simulink model "Totem_PSFB_Charger"  (R2022a)
settings: Solver=ode4  StartTime=0.0  StopTime=1  FixedStep=1e-7  RelTol=1e-3
undefined symbols (not defined in the file): C_PSFB, C_totem, fs_PFC, Gci_inf, Gcinf, Gcv_inf, Gcvinf, H, H_PSFB, kx, L_PSFB, L_totem, Rsense, Rsense_PSFB, Vm, wL, wLi_PSFB, wLv_PSFB, wLvv
libraries: spsMosfetLib x9, spsDiodeLib x8, spsSeriesRLCBranchLib x8, spsVoltageMeasurementLib x4, spsCurrentMeasurementLib x2, spsACVoltageSourceLib x1, hdlsllib x1, spsLinearTransformerLib x1, spsDCVoltageSourceLib x1, spsRMSLib x1, simulink x1, spspowerguiLib x1
settings Model: Creator=Aditya Bhalotia  LastModifiedBy=Aditya Bhalotia
settings DataIOCC: ReturnWorkspaceOutputs=off

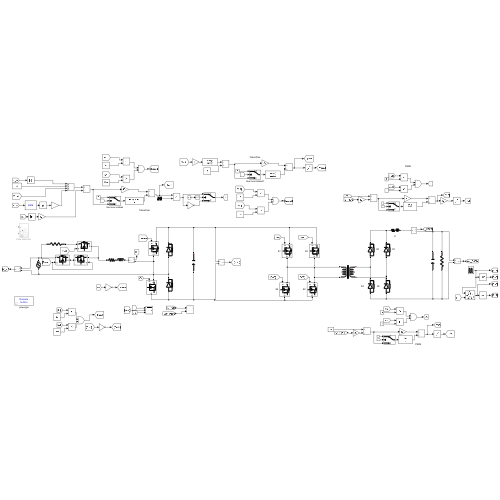
[thumbnail: Simulink's stored preview of the top-level diagram]
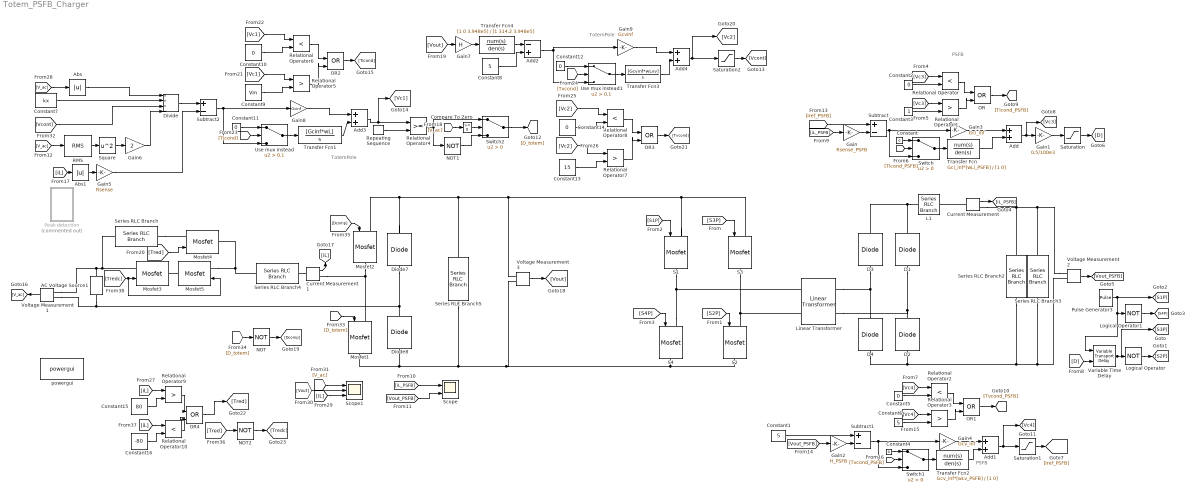
== system Totem_PSFB_Charger ==
  note: TotemPole
  note: PSFB
  note: PSFB
  note: TotemPole
  AC Voltage Source1 : spsACVoltageSourceLib/AC Voltage Source  Amplitude=265*sqrt(2)  Phase=0  Frequency=65  SampleTime=0  Measurements=None  BusType=swing  Pref=10e3  Qref=0  Qmin=-inf  Qmax=+inf
  Abs : Abs  SaturateOnIntegerOverflow=off
  Abs1 : Abs  SaturateOnIntegerOverflow=off
  Add{,1,3..4} (4 alike) : Sum
  Add2 : Sum  Inputs=-+
  Compare To Zero : hdlsllib/Logic and Bit Operations/Compare To Zero  relop=>=  OutDataTypeStr=boolean
      settings: SourceProductBaseCode=SL
  Constant{,2,4..5,10..12,14} (8 alike) : Constant  Value=0
  Constant1 : Constant  Value=5
  Constant13 : Constant  Value=15
  Constant15 : Constant  Value=80
  Constant16 : Constant  Value=-80
  Constant3 : Constant
  Constant6 : Constant  Value=5
  Constant7 : Constant  Value=kx
  Constant8 : Constant  Value=5
  Constant9 : Constant  Value=Vm
  Current Measurement : spsCurrentMeasurementLib/Current Measurement  PhasorSimulation=off  OutputType=Complex  PSBequivalent=0
  Current Measurement1 : spsCurrentMeasurementLib/Current Measurement  PhasorSimulation=off  OutputType=Complex  PSBequivalent=0
  D{1..4} (4 alike) : spsDiodeLib/Diode  Ron=0.001  Lon=0  Vf=1  IC=0  UseSnubber=0  Rs=500e6  Cs=1e-15  Measurements=off
  Diode7 : spsDiodeLib/Diode  Ron=0.001  Lon=0  Vf=0  IC=0  UseSnubber=0  Rs=50e3  Cs=inf  Measurements=off
  Diode8 : spsDiodeLib/Diode  Ron=0.001  Lon=0  Vf=0  IC=0  UseSnubber=0  Rs=50e3  Cs=inf  Measurements=off
  Divide : Product  Inputs=***/
  Gain : Gain  Gain=Rsense_PSFB
  Gain1 : Gain  Gain=0.5/100e3
  Gain2 : Gain  Gain=H_PSFB
  Gain3 : Gain  Gain=Gci_inf
  Gain4 : Gain  Gain=Gcv_inf
  Gain5 : Gain  Gain=Rsense
  Gain6 : Gain  Gain=2
  Gain7 : Gain  Gain=H
  Gain8 : Gain  Gain=Gcinf
  Gain9 : Gain  Gain=Gcvinf
  L1 : spsSeriesRLCBranchLib/Series RLC Branch  LConnTagsString=__new0  RConnTagsString=__new0  BranchType=RL  Resistance=0.1  Inductance=L_PSFB  SetiL0=off  InitialCurrent=0  Capacitance=1e-6  Setx0=off  InitialVoltage=0  Measurements=Branch current
  Linear Transformer : spsLinearTransformerLib/Linear Transformer  UNITS=SI  NominalPower=[50e2 100e3]  winding1=[400 0.01 0]  winding2=[400 0.01 0]  ThreeWindings=off  winding3=[3.15e+05 0.7938 0.084225]  RmLm=[1.0804e5 28e-3]  Measurements=None  DataType=on
  Logical Operator : Logic  Operator=NOT  AllPortsSameDT=off  OutDataTypeStr=boolean
  Logical Operator1 : Logic  Operator=NOT  AllPortsSameDT=off  OutDataTypeStr=boolean
  Mosfet{1..5} (5 alike) : spsMosfetLib/Mosfet  Ron=0.0001  Lon=0  Rd=0.0001  Vfd=0  IC=0  Rs=50e4  Cs=inf  Measurements=off
  NOT : Logic  Operator=NOT  IconShape=distinctive  AllPortsSameDT=off  OutDataTypeStr=boolean
  NOT1 : Logic  Operator=NOT  IconShape=distinctive  AllPortsSameDT=off  OutDataTypeStr=boolean
  NOT2 : Logic  Operator=NOT  IconShape=distinctive  AllPortsSameDT=off  OutDataTypeStr=boolean
  OR{,1..4} (5 alike) : Logic  Operator=OR  IconShape=distinctive  AllPortsSameDT=off  OutDataTypeStr=boolean
  Peak detection : Subsystem  Commented=on
  Pulse Generator3 : DiscretePulseGenerator  PulseType=Time based  Period=10e-6  PulseWidth=50
  RMS : spsRMSLib/RMS  TrueRMS=off  Freq=65  RMSInit=220  Ts=0
  Relational Operator{,2,6,8,10} (5 alike) : RelationalOperator  Operator=<  OutDataTypeStr=boolean  RndMeth=Simplest  InputSameDT=off
  Relational Operator{1,3,5,7,9} (5 alike) : RelationalOperator  Operator=>  OutDataTypeStr=boolean  RndMeth=Simplest  InputSameDT=off
  Relational Operator4 : RelationalOperator  OutDataTypeStr=boolean  RndMeth=Simplest  InputSameDT=off
  Repeating Sequence : simulink/Sources/Repeating Sequence  rep_seq_t=[0 1/fs_PFC]  rep_seq_y=[0 Vm]
  S{1..4} (4 alike) : spsMosfetLib/Mosfet  Ron=0.001  Lon=0  Rd=0.01  Vfd=0  IC=0  Rs=1e5  Cs=inf  Measurements=off
  Saturation : Saturate  UpperLimit=5e-6  LowerLimit=0
  Saturation1 : Saturate  UpperLimit=5  LowerLimit=0
  Saturation2 : Saturate  UpperLimit=15  LowerLimit=0
  Scope : Scope  NumInputPorts=2
  Scope1 : Scope  NumInputPorts=3
  Series RLC Branch : spsSeriesRLCBranchLib/Series RLC Branch  LConnTagsString=__new0  RConnTagsString=__new0  BranchType=R  Resistance=5  Inductance=1e-3  SetiL0=off  InitialCurrent=0  Capacitance=1e-6  Setx0=off  InitialVoltage=0  Measurements=None
  Series RLC Branch2 : spsSeriesRLCBranchLib/Series RLC Branch  LConnTagsString=__new0  RConnTagsString=__new0  BranchType=C  Resistance=1  Inductance=1e-3  SetiL0=off  InitialCurrent=0  Capacitance=C_PSFB  Setx0=off  InitialVoltage=0  Measurements=None
  Series RLC Branch3 : spsSeriesRLCBranchLib/Series RLC Branch  LConnTagsString=__new0  RConnTagsString=__new0  BranchType=R  Resistance=313.6  Inductance=1e-3  SetiL0=off  InitialCurrent=0  Capacitance=1e-6  Setx0=off  InitialVoltage=0  Measurements=None
  Series RLC Branch4 : spsSeriesRLCBranchLib/Series RLC Branch  LConnTagsString=__new0  RConnTagsString=__new0  BranchType=RL  Resistance=0.2  Inductance=L_totem  SetiL0=off  InitialCurrent=0  Capacitance=1e-6  Setx0=off  InitialVoltage=0  Measurements=None
  Series RLC Branch5 : spsSeriesRLCBranchLib/Series RLC Branch  LConnTagsString=__new0  RConnTagsString=__new0  BranchType=C  Resistance=1  Inductance=1e-3  SetiL0=off  InitialCurrent=0  Capacitance=C_totem  Setx0=off  InitialVoltage=0  Measurements=None
  Square : Math  Operator=square  OutputSignalType=real
  Subtract : Sum  Inputs=+-
  Subtract1 : Sum  Inputs=+-
  Subtract2 : Sum  Inputs=+-
  Switch : Switch  Criteria=u2 > Threshold  SaturateOnIntegerOverflow=off  InputSameDT=off
  Switch1 : Switch  Criteria=u2 > Threshold  SaturateOnIntegerOverflow=off  InputSameDT=off
  Switch2 : Switch  Criteria=u2 > Threshold  SaturateOnIntegerOverflow=off  InputSameDT=off
  Transfer Fcn : TransferFcn  Numerator=Gci_inf*[wLi_PSFB]  Denominator=[1 0]
  Transfer Fcn1 : TransferFcn  Numerator=[Gcinf*wL]  Denominator=[1 0]
  Transfer Fcn2 : TransferFcn  Numerator=Gcv_inf*[wLv_PSFB]  Denominator=[1 0]
  Transfer Fcn3 : TransferFcn  Numerator=[Gcvinf*wLvv]  Denominator=[1 0]
  Transfer Fcn4 : TransferFcn  Numerator=[1 0 3.948e5]  Denominator=[1 314.2 3.948e5]
  Use mux instead : Switch  Criteria=u2 > Threshold  Threshold=0.1  SaturateOnIntegerOverflow=off  InputSameDT=off
  Use mux instead1 : Switch  Criteria=u2 > Threshold  Threshold=0.1  SaturateOnIntegerOverflow=off  InputSameDT=off
  Variable Time Delay : VariableTransportDelay  MaximumDelay=5.1e-6
  Voltage Measurement1 : spsVoltageMeasurementLib/Voltage Measurement  PhasorSimulation=off  OutputType=Complex  PSBequivalent=0
  Voltage Measurement2 : spsVoltageMeasurementLib/Voltage Measurement  PhasorSimulation=off  OutputType=Complex  PSBequivalent=0
  Voltage Measurement3 : spsVoltageMeasurementLib/Voltage Measurement  PhasorSimulation=off  OutputType=Complex  PSBequivalent=0
  powergui : spspowerguiLib/powergui  Priority=1  SimulationMode=Discrete  SampleTime=1e-8  frequency=60  Iterations=50  frequencyindice=0  Pbase=100e6  ErrMax=1e-4  UnitsV=kV  UnitsW=MW  buscounter=0  FunctionMessages=off  echomessages=off  EnableUseOfTLC=off  CurrentSourceSwitches=off  DisableSnubberDevices=off  DisableRonSwitches=off  DisableVfSwitches=off  DisplayEquations=off  AutomaticDiscreteSolvers=off  SolverType=Tustin/Backward Euler (TBE)  Interpol=off  ExternalGateDelay=off  methode=off  Ts=100  x0status=blocks  SPID=on  SwTol=0  HookPort=off  NonlinearTolerance=1e-4  nMaxIteration=100  ContinueOnMaxIteration=off  RestoreLinks=warning  ResistiveCurrentMeasurement=off  Frange=[0:2:500]  Ylog=off  Xlog=on  ShowGrid=off  save=off  variable=ZData  structure=0  ZoomFFT=off  StartTime=0.0  cycles=1  DisplayStyle=1  fundamental=60  FreqAxis=off  MaxFrequency=1000  frequencyindicesteady=1  RmsSteady=1  display=off
  wires:
  Relational Operator3/1 -> OR1/2
  [Tvcond_PSFB] -> Switch1/2
  [Ticond_PSFB] -> Switch/2
  OR/1 -> [Ticond_PSFB]
  Constant3/1 -> Relational Operator1/2
  [Vc3] -> Relational Operator1/1
  [Vc3] -> Relational Operator/1
  Constant5/1 -> Relational Operator2/2
  Switch1/1 -> Transfer Fcn2/1
  OR1/1 -> [Tvcond_PSFB]
  Relational Operator/1 -> OR/1
  Subtract1/1 -> Switch1/3, Gain4/1
  Constant2/1 -> Relational Operator/2
  Add/1 -> Gain1/1, [Vc3]
  Switch/1 -> Transfer Fcn/1
  Gain3/1 -> Add/1
  Constant/1 -> Switch/1
  Relational Operator2/1 -> OR1/1
  [Vc4] -> Relational Operator2/1
  Transfer Fcn/1 -> Add/2
  Logical Operator1/1 -> [S4P]
  Gain1/1 -> Saturation/1
  Gain/1 -> Subtract/2
  Add1/1 -> Saturation1/1, [Vc4]
  [D] -> Variable Time Delay/2
  Voltage Measurement2/1 -> [Vout_PSFB]
  [S2P] -> S2/1
  [iL_PSFB] -> Gain/1
  [Iref_PSFB] -> Subtract/1
  [S1P] -> S1/1
  Pulse Generator3/1 -> Variable Time Delay/1, Logical Operator1/1, [S1P]
  [S4P] -> S4/1
  Variable Time Delay/1 -> [S3P], Logical Operator/1
  Constant6/1 -> Relational Operator3/2
  [Vc4] -> Relational Operator3/1
  Current Measurement/1 -> [iL_PSFB]
  Relational Operator1/1 -> OR/2
  Gain2/1 -> Subtract1/2
  Subtract/1 -> Switch/3, Gain3/1
  [Vout_PSFB] -> Scope/2
  Constant1/1 -> Subtract1/1
  Saturation1/1 -> [Iref_PSFB]
  Saturation/1 -> [D]
  [Vout_PSFB] -> Gain2/1
  [S3P] -> S3/1
  [iL_PSFB] -> Scope/1
  Gain4/1 -> Add1/1
  Constant4/1 -> Switch1/1
  Logical Operator/1 -> [S2P]
  Transfer Fcn2/1 -> Add1/2
  Saturation2/1 -> [Vcont]
  Constant12/1 -> Use mux instead1/1
  Gain8/1 -> Add3/1
  Add4/1 -> Saturation2/1, [Vc2]
  [Vc2] -> Relational Operator7/1
  [V_ac] -> RMS/1
  Transfer Fcn3/1 -> Add4/2
  Square/1 -> Gain6/1
  Add3/1 -> Relational Operator4/1, [Vc1]
  OR3/1 -> [Tvcond]
  Subtract2/1 -> Gain8/1, Use mux instead/3
  Constant13/1 -> Relational Operator7/2
  Gain9/1 -> Add4/1
  [Vc2] -> Relational Operator8/1
  Relational Operator8/1 -> OR3/1
  Relational Operator5/1 -> OR2/2
  Gain6/1 -> Divide/4
  [Dcomp] -> Mosfet2/1
  [Vout] -> Scope1/2
  Relational Operator7/1 -> OR3/2
  Use mux instead/1 -> Transfer Fcn1/1
  [Tvcond] -> Use mux instead1/2
  Use mux instead1/1 -> Transfer Fcn3/1
  Constant14/1 -> Relational Operator8/2
  [Ticond] -> Use mux instead/2
  [Vc1] -> Relational Operator6/1
  OR2/1 -> [Ticond]
  Constant10/1 -> Relational Operator6/2
  [Vcont] -> Divide/3
  Divide/1 -> Subtract2/1
  Compare To Zero/1 -> Switch2/2
  Constant9/1 -> Relational Operator5/2
  [Vc1] -> Relational Operator5/1
  Constant11/1 -> Use mux instead/1
  Transfer Fcn1/1 -> Add3/2
  [D_totem] -> Mosfet1/1
  Constant8/1 -> Add2/2
  Gain5/1 -> Subtract2/2
  Relational Operator4/1 -> NOT1/1, Switch2/1
  RMS/1 -> Square/1
  Abs1/1 -> Gain5/1
  NOT1/1 -> Switch2/3
  [Vout] -> Gain7/1
  [D_totem] -> NOT/1
  [V_ac] -> Compare To Zero/1
  NOT/1 -> [Dcomp]
  Voltage Measurement1/1 -> [V_ac]
  Current Measurement1/1 -> [iL]
  Gain7/1 -> Transfer Fcn4/1
  Relational Operator6/1 -> OR2/1
  Switch2/1 -> [D_totem]
  [iL] -> Abs1/1
  [V_ac] -> Abs/1
  Abs/1 -> Divide/1
  [iL] -> Scope1/3
  Voltage Measurement3/1 -> [Vout]
  Repeating Sequence/1 -> Relational Operator4/2
  [V_ac] -> Scope1/1
  Constant7/1 -> Divide/2
  [Tred] -> Mosfet4/1
  OR4/1 -> [Tred]
  [Tred] -> NOT2/1
  Constant16/1 -> Relational Operator10/2
  Constant15/1 -> Relational Operator9/2
  [iL] -> Relational Operator9/1
  [iL] -> Relational Operator10/1
  Relational Operator9/1 -> OR4/1
  NOT2/1 -> [Tredc]
  Relational Operator10/1 -> OR4/2
  [Tredc] -> Mosfet5/1, Mosfet3/1
  Transfer Fcn4/1 -> Add2/1
  Add2/1 -> Gain9/1, Use mux instead1/3
  connections:
  S2/LConn1 -- S3/RConn1 -- Linear Transformer/LConn2
  D2/RConn1 -- D1/LConn1 -- Linear Transformer/RConn2
  S4/LConn1 -- S1/RConn1 -- Linear Transformer/LConn1
  Voltage Measurement2/LConn1 -- Series RLC Branch3/LConn1 -- Current Measurement/RConn1 -- Series RLC Branch2/LConn1
  Series RLC Branch3/RConn1 -- D4/LConn1 -- D2/LConn1 -- Series RLC Branch2/RConn1 -- Voltage Measurement2/LConn2
  Diode8/LConn1 -- S2/RConn1 -- S4/RConn1 -- Voltage Measurement3/LConn2 -- Series RLC Branch5/RConn1 -- Mosfet1/RConn1
  Linear Transformer/RConn1 -- D4/RConn1 -- D3/LConn1
  Diode7/RConn1 -- Series RLC Branch5/LConn1 -- Voltage Measurement3/LConn1 -- S3/LConn1 -- S1/LConn1 -- Mosfet2/LConn1
  L1/LConn1 -- D3/RConn1 -- D1/RConn1
  Current Measurement/LConn1 -- L1/RConn1
  Series RLC Branch/LConn1 -- Mosfet3/LConn1 -- Voltage Measurement1/LConn1 -- AC Voltage Source1/RConn1
  Mosfet1/LConn1 -- Current Measurement1/RConn1 -- Mosfet2/RConn1
  Voltage Measurement1/LConn2 -- Diode8/RConn1 -- Diode7/LConn1 -- AC Voltage Source1/LConn1
  Series RLC Branch4/RConn1 -- Current Measurement1/LConn1
  Series RLC Branch4/LConn1 -- Mosfet4/RConn1 -- Mosfet5/LConn1
  Series RLC Branch/RConn1 -- Mosfet4/LConn1
  Mosfet5/RConn1 -- Mosfet3/RConn1

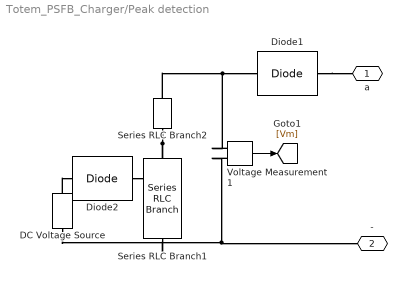
== system Totem_PSFB_Charger/Peak detection ==
  DC Voltage Source : spsDCVoltageSourceLib/DC Voltage Source  Amplitude=1  Measurements=None
  Diode1 : spsDiodeLib/Diode  Ron=0.001  Lon=0  Vf=0  IC=0  UseSnubber=0  Rs=inf  Cs=inf  Measurements=off
  Diode2 : spsDiodeLib/Diode  Ron=0.001  Lon=0  Vf=0  IC=0  UseSnubber=0  Rs=inf  Cs=inf  Measurements=off
  Series RLC Branch1 : spsSeriesRLCBranchLib/Series RLC Branch  LConnTagsString=__new0  RConnTagsString=__new0  BranchType=C  Resistance=1  Inductance=1e-3  SetiL0=off  InitialCurrent=0  Capacitance=100e-6  Setx0=on  InitialVoltage=0  Measurements=None
  Series RLC Branch2 : spsSeriesRLCBranchLib/Series RLC Branch  LConnTagsString=__new0  RConnTagsString=__new0  BranchType=R  Resistance=2e-3  Inductance=1e-3  SetiL0=off  InitialCurrent=0  Capacitance=1e-6  Setx0=off  InitialVoltage=0  Measurements=Branch voltage
  Voltage Measurement1 : spsVoltageMeasurementLib/Voltage Measurement  PhasorSimulation=off  OutputType=Complex  PSBequivalent=0
  a : PMIOPort  Side=Left
  - : PMIOPort  Port=2  Side=Left
  wires:
  Voltage Measurement1/1 -> [Vm]
  connections:
  Voltage Measurement1/LConn2 -- DC Voltage Source/LConn1 -- Series RLC Branch1/RConn1 -- -/RConn1
  Diode1/LConn1 -- a/RConn1
  Series RLC Branch2/LConn1 -- Voltage Measurement1/LConn1 -- Diode1/RConn1
  DC Voltage Source/RConn1 -- Diode2/LConn1
  Series RLC Branch2/RConn1 -- Diode2/RConn1 -- Series RLC Branch1/LConn1
